simulink model "simulateAICENRobotInGazebo"  (R2022a)
settings: Solver=FixedStepAuto  StartTime=0.0  StopTime=inf  RelTol=1e-3
model workspace (MAT data in the model file):
  start = [2 8]
undefined symbols (not defined in the file or in its folder): avoidCollisionDistance, chargingStn, duration, effort, index, joint_name, left_wheel_clone_hinge, left_wheel_hinge, loadingStn, logicalMap, model_name, right_wheel_clone_hinge, right_wheel_hinge, scoutmini3, unloadingStn
libraries: robotgazebolib x19, robotalgslib x1, robotcorelib x1
settings Model: ParameterArgumentNames=start  Creator=The MathWorks, Inc.  LastModifiedBy=USER
settings SolverCC: AlgebraicLoopSolver=TrustRegion
settings DebuggingCC: UnconnectedInputMsg=warning  UnconnectedOutputMsg=warning  UnconnectedLineMsg=warning  ModelReferenceExtraNoncontSigs=none  SymbolicDimsDataTypeCodeGenerationDiagnostic=none  SFMachineParentedDataDiag=warning
settings RTWCC: DLArmComputeVersion=19.05

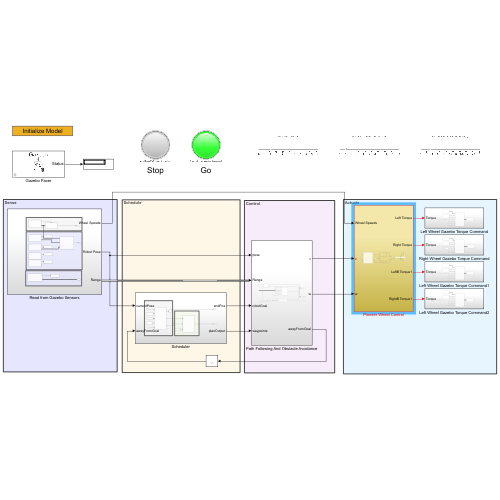
[thumbnail: Simulink's stored preview of the top-level diagram]
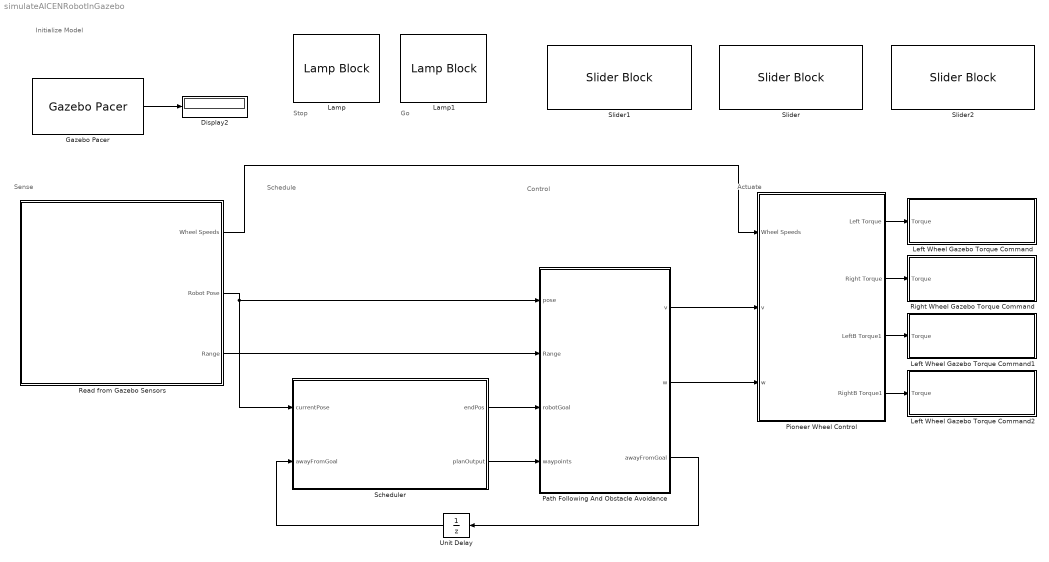
== system simulateAICENRobotInGazebo ==
  note: Actuate
  note: Control
  note: Schedule
  note: Sense
  note: Initialize Model
  note: Stop
  note: Go
  Display2 : Display
  Gazebo Pacer : robotgazebolib/Gazebo Pacer  ResetBehavior=Reset Gazebo simulation time and scene  SampleTime=0.01
      settings: SourceProductBaseCode=RO
  Lamp : LampBlock  LabelPosition=Bottom
  Lamp1 : LampBlock  LabelPosition=Bottom
  Left Wheel Gazebo Torque Command : Subsystem
  Left Wheel Gazebo Torque Command1 : Subsystem
  Left Wheel Gazebo Torque Command2 : Subsystem
  Path Following And Obstacle Avoidance : Subsystem
  Pioneer Wheel Control : Subsystem
  Read from Gazebo Sensors : Subsystem
  Right Wheel Gazebo Torque Command : Subsystem
  Scheduler : Subsystem
  Slider : SliderBlock  ScaleMax=10
  Slider1 : SliderBlock  ScaleMax=10
  Slider2 : SliderBlock  ScaleMax=5
  Unit Delay : UnitDelay  InitialCondition=1  SampleTime=-1  HasFrameUpgradeWarning=on
  wires:
  Read from Gazebo Sensors/2(Robot Pose) -> Scheduler/1(currentPose), Path Following And Obstacle Avoidance/1(pose)
  Pioneer Wheel Control/1(Left Torque) -> Left Wheel Gazebo Torque Command/1(Torque)
  Pioneer Wheel Control/2(Right Torque) -> Right Wheel Gazebo Torque Command/1(Torque)
  Read from Gazebo Sensors/1(Wheel Speeds) -> Pioneer Wheel Control/1(Wheel Speeds)
  Read from Gazebo Sensors/3(Range) -> Path Following And Obstacle Avoidance/2(Range)
  Path Following And Obstacle Avoidance/2(w) -> Pioneer Wheel Control/3(w)
  Gazebo Pacer/1 -> Display2/1
  Path Following And Obstacle Avoidance/3(awayFromGoal) -> Unit Delay/1
  Scheduler/1(endPos) -> Path Following And Obstacle Avoidance/3(robotGoal)
  Scheduler/2(planOutput) -> Path Following And Obstacle Avoidance/4(waypoints)
  Unit Delay/1 -> Scheduler/2(awayFromGoal)
  Path Following And Obstacle Avoidance/1(v) -> Pioneer Wheel Control/2(v)
  Pioneer Wheel Control/3(LeftB Torque1) -> Left Wheel Gazebo Torque Command1/1(Torque)
  Pioneer Wheel Control/4(RightB Torque1) -> Left Wheel Gazebo Torque Command2/1(Torque)

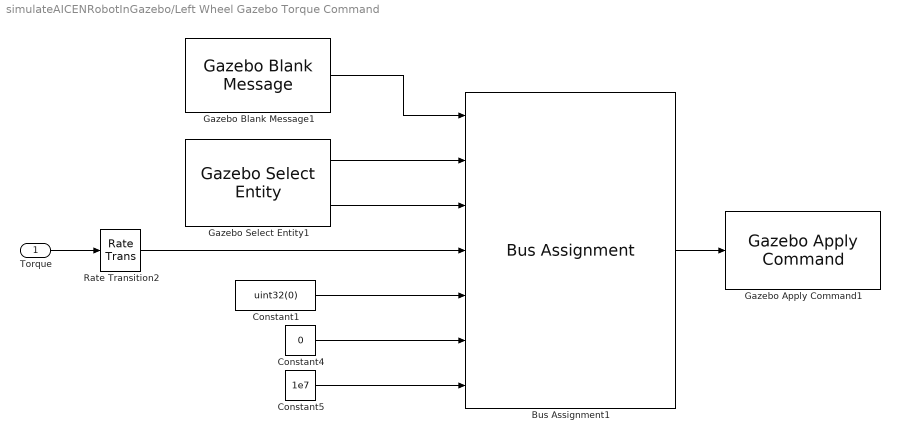
== system simulateAICENRobotInGazebo/Left Wheel Gazebo Torque Command ==
  Torque : Inport
  Bus Assignment1 : BusAssignment  AssignedSignals=model_name,joint_name,effort,index,duration.seconds,duration.nano_seconds
  Constant1 : Constant  Value=uint32(0)
  Constant4 : Constant  Value=0
  Constant5 : Constant  Value=1e7
  Gazebo Apply Command1 : robotgazebolib/Gazebo Apply Command  cmdType=ApplyJointTorque  sampleTime=0.01
      settings: SourceProductBaseCode=RO
  Gazebo Blank Message1 : robotgazebolib/Gazebo Blank Message  msgType=ApplyJointTorque  sampleTime=0.01  busName='Gazebo_SL_Bus_gazebo_msgs_ApplyJointTorque'
      settings: SourceProductBaseCode=RO
  Gazebo Select Entity1 : robotgazebolib/Gazebo Select Entity  modelElemName=scoutmini3/left_wheel_hinge  outputArraySize=128  OutputLabel=Joint  SelectType=Joint
      settings: SourceProductBaseCode=RO
  Rate Transition2 : RateTransition
  wires:
  Bus Assignment1/1 -> Gazebo Apply Command1/1
  Constant5/1 -> Bus Assignment1/7
  Gazebo Blank Message1/1 -> Bus Assignment1/1
  Gazebo Select Entity1/2 -> Bus Assignment1/3
  Gazebo Select Entity1/1 -> Bus Assignment1/2
  Torque/1 -> Rate Transition2/1
  Constant4/1 -> Bus Assignment1/6
  Rate Transition2/1 -> Bus Assignment1/4
  Constant1/1 -> Bus Assignment1/5

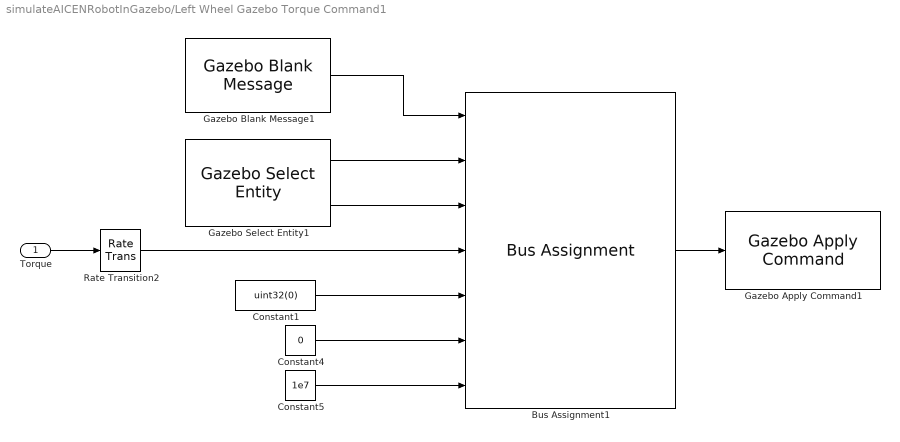
== system simulateAICENRobotInGazebo/Left Wheel Gazebo Torque Command1 ==
  Torque : Inport
  Bus Assignment1 : BusAssignment  AssignedSignals=model_name,joint_name,effort,index,duration.seconds,duration.nano_seconds
  Constant1 : Constant  Value=uint32(0)
  Constant4 : Constant  Value=0
  Constant5 : Constant  Value=1e7
  Gazebo Apply Command1 : robotgazebolib/Gazebo Apply Command  cmdType=ApplyJointTorque  sampleTime=0.01
      settings: SourceProductBaseCode=RO
  Gazebo Blank Message1 : robotgazebolib/Gazebo Blank Message  msgType=ApplyJointTorque  sampleTime=0.01  busName='Gazebo_SL_Bus_gazebo_msgs_ApplyJointTorque'
      settings: SourceProductBaseCode=RO
  Gazebo Select Entity1 : robotgazebolib/Gazebo Select Entity  modelElemName=scoutmini3/left_wheel_clone_hinge  outputArraySize=128  OutputLabel=Joint  SelectType=Joint
      settings: SourceProductBaseCode=RO
  Rate Transition2 : RateTransition
  wires:
  Bus Assignment1/1 -> Gazebo Apply Command1/1
  Constant5/1 -> Bus Assignment1/7
  Gazebo Blank Message1/1 -> Bus Assignment1/1
  Gazebo Select Entity1/2 -> Bus Assignment1/3
  Gazebo Select Entity1/1 -> Bus Assignment1/2
  Torque/1 -> Rate Transition2/1
  Constant4/1 -> Bus Assignment1/6
  Rate Transition2/1 -> Bus Assignment1/4
  Constant1/1 -> Bus Assignment1/5

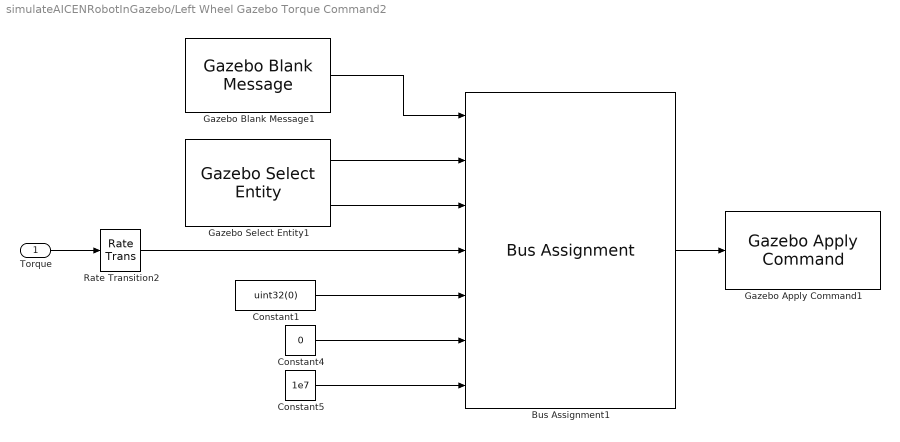
== system simulateAICENRobotInGazebo/Left Wheel Gazebo Torque Command2 ==
  Torque : Inport
  Bus Assignment1 : BusAssignment  AssignedSignals=model_name,joint_name,effort,index,duration.seconds,duration.nano_seconds
  Constant1 : Constant  Value=uint32(0)
  Constant4 : Constant  Value=0
  Constant5 : Constant  Value=1e7
  Gazebo Apply Command1 : robotgazebolib/Gazebo Apply Command  cmdType=ApplyJointTorque  sampleTime=0.01
      settings: SourceProductBaseCode=RO
  Gazebo Blank Message1 : robotgazebolib/Gazebo Blank Message  msgType=ApplyJointTorque  sampleTime=0.01  busName='Gazebo_SL_Bus_gazebo_msgs_ApplyJointTorque'
      settings: SourceProductBaseCode=RO
  Gazebo Select Entity1 : robotgazebolib/Gazebo Select Entity  modelElemName=scoutmini3/right_wheel_clone_hinge  outputArraySize=128  OutputLabel=Joint  SelectType=Joint
      settings: SourceProductBaseCode=RO
  Rate Transition2 : RateTransition
  wires:
  Bus Assignment1/1 -> Gazebo Apply Command1/1
  Constant5/1 -> Bus Assignment1/7
  Gazebo Blank Message1/1 -> Bus Assignment1/1
  Gazebo Select Entity1/2 -> Bus Assignment1/3
  Gazebo Select Entity1/1 -> Bus Assignment1/2
  Torque/1 -> Rate Transition2/1
  Constant4/1 -> Bus Assignment1/6
  Rate Transition2/1 -> Bus Assignment1/4
  Constant1/1 -> Bus Assignment1/5

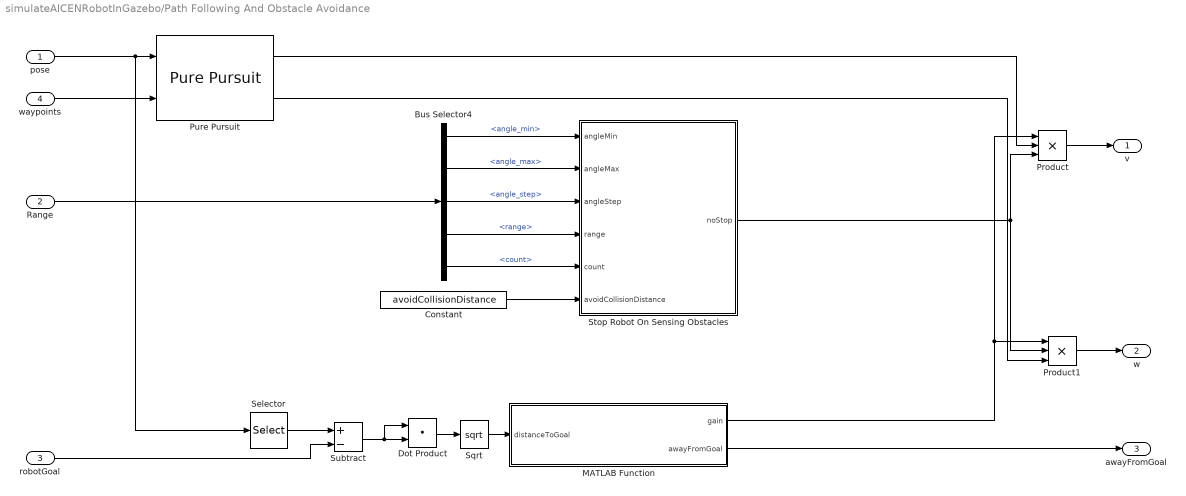
== system simulateAICENRobotInGazebo/Path Following And Obstacle Avoidance ==
  pose : Inport
  Range : Inport  Port=2
  robotGoal : Inport  Port=3
  waypoints : Inport  Port=4
  Bus Selector4 : BusSelector  OutputSignals=angle_min,angle_max,angle_step,range,count
  Constant : Constant  Value=avoidCollisionDistance
  Dot Product : DotProduct  OutDataTypeStr=Inherit: Inherit via internal rule
  MATLAB Function : MATLAB Function  TreatAsAtomicUnit=on
  Product : Product  Inputs=3
  Product1 : Product  Inputs=3
  Pure Pursuit : robotalgslib/Pure Pursuit  DesiredLinearVelocity=0.8  MaxAngularVelocity=1  LookaheadDistance=1  TargetDirPort=off  SimulateUsing=Code generation
  Selector : Selector  InputPortWidth=3  IndexOptions=Index vector (dialog)  Indices=[1 2]  OutputSizes=1
  Sqrt : Sqrt
  Stop Robot On Sensing Obstacles : MATLAB Function  TreatAsAtomicUnit=on
  Subtract : Sum  Inputs=+-
  v : Outport
  w : Outport  Port=2
  awayFromGoal : Outport  Port=3
  wires:
  Product1/1 -> w/1
  Product/1 -> v/1
  Stop Robot On Sensing Obstacles/1(noStop) -> Product/3, Product1/2
  Pure Pursuit/1 -> Product/2
  Pure Pursuit/2 -> Product1/3
  MATLAB Function/1(gain) -> Product/1, Product1/1
  Bus Selector4/4 -> Stop Robot On Sensing Obstacles/4(range)  "<range>"
  Range/1 -> Bus Selector4/1
  Constant/1 -> Stop Robot On Sensing Obstacles/6(avoidCollisionDistance)
  Bus Selector4/5 -> Stop Robot On Sensing Obstacles/5(count)  "<count>"
  Bus Selector4/1 -> Stop Robot On Sensing Obstacles/1(angleMin)  "<angle_min>"
  Bus Selector4/2 -> Stop Robot On Sensing Obstacles/2(angleMax)  "<angle_max>"
  Bus Selector4/3 -> Stop Robot On Sensing Obstacles/3(angleStep)  "<angle_step>"
  Sqrt/1 -> MATLAB Function/1(distanceToGoal)
  Subtract/1 -> Dot Product/1, Dot Product/2
  Selector/1 -> Subtract/1
  Dot Product/1 -> Sqrt/1
  robotGoal/1 -> Subtract/2
  MATLAB Function/2(awayFromGoal) -> awayFromGoal/1
  pose/1 -> Selector/1, Pure Pursuit/1
  waypoints/1 -> Pure Pursuit/2

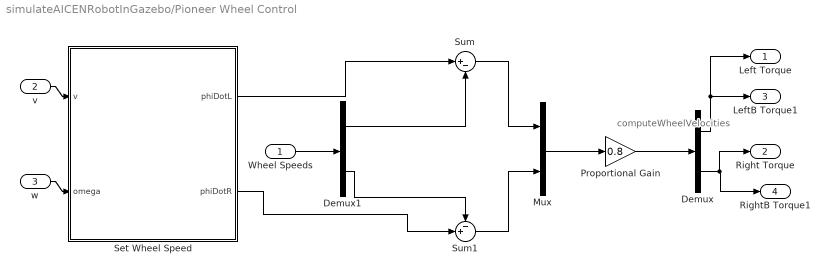
== system simulateAICENRobotInGazebo/Pioneer Wheel Control ==
  note: computeWheelVelocities
  Wheel Speeds : Inport
  v : Inport  Port=2
  w : Inport  Port=3
  Demux : Demux  Outputs=2
  Demux1 : Demux  Outputs=2
  Mux : Mux  Inputs=2
  Proportional Gain : Gain  Gain=0.8
  Set Wheel Speed : MATLAB Function  TreatAsAtomicUnit=on
  Sum : Sum  Inputs=|+-
  Sum1 : Sum  Inputs=-+|
  Left Torque : Outport
  Right Torque : Outport  Port=2
  LeftB Torque1 : Outport  Port=3
  RightB Torque1 : Outport  Port=4
  wires:
  Sum1/1 -> Mux/2
  Set Wheel Speed/1(phiDotL) -> Sum/1
  Sum/1 -> Mux/1
  Mux/1 -> Proportional Gain/1
  Proportional Gain/1 -> Demux/1
  Wheel Speeds/1 -> Demux1/1
  Demux1/1 -> Sum/2
  Set Wheel Speed/2(phiDotR) -> Sum1/2
  Demux1/2 -> Sum1/1
  v/1 -> Set Wheel Speed/1(v)
  w/1 -> Set Wheel Speed/2(omega)
  Demux/2 -> Right Torque/1, RightB Torque1/1
  Demux/1 -> LeftB Torque1/1, Left Torque/1

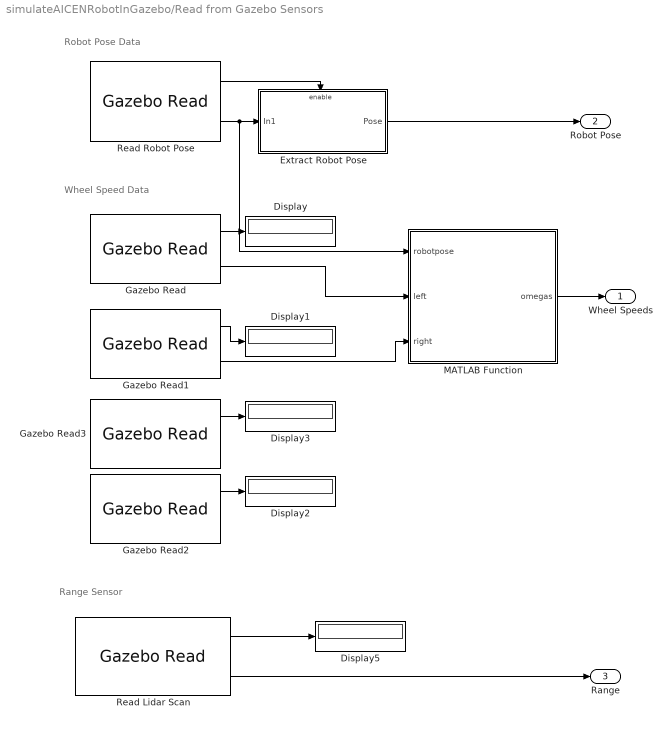
== system simulateAICENRobotInGazebo/Read from Gazebo Sensors ==
  note: Robot Pose Data
  note: Wheel Speed Data
  note: Range Sensor
  Display{,1..3,5} (5 alike) : Display
  Extract Robot Pose : Subsystem
  Gazebo Read : robotgazebolib/Gazebo Read  topicSource=Specify your own  topic=/gazebo/ground_truth/world_pose/scoutmini3/left_wheel  messageType=gazebo_msgs/Pose  sampleTime=0.01
      settings: SourceProductBaseCode=RO
  Gazebo Read1 : robotgazebolib/Gazebo Read  topicSource=Specify your own  topic=/gazebo/ground_truth/world_pose/scoutmini3/right_wheel  messageType=gazebo_msgs/Pose  sampleTime=0.01
      settings: SourceProductBaseCode=RO
  Gazebo Read2 : robotgazebolib/Gazebo Read  topicSource=Specify your own  topic=/gazebo/ground_truth/world_pose/scoutmini3/right_wheel_clone  messageType=gazebo_msgs/Pose  sampleTime=0.01
      settings: SourceProductBaseCode=RO
  Gazebo Read3 : robotgazebolib/Gazebo Read  topicSource=Specify your own  topic=/gazebo/ground_truth/world_pose/scoutmini3/left_wheel_clone  messageType=gazebo_msgs/Pose  sampleTime=0.01
      settings: SourceProductBaseCode=RO
  MATLAB Function : MATLAB Function  TreatAsAtomicUnit=on
  Read Lidar Scan : robotgazebolib/Gazebo Read  topicSource=Specify your own  topic=/gazebo/default/scoutmini3/hokuyo/link/laser/scan  messageType=gazebo_msgs/LaserScan  sampleTime=0.01
      settings: SourceProductBaseCode=RO
  Read Robot Pose : robotgazebolib/Gazebo Read  topicSource=Specify your own  topic=/gazebo/ground_truth/world_pose/scoutmini3/chassis  messageType=gazebo_msgs/Pose  sampleTime=0.01
      settings: SourceProductBaseCode=RO
  Wheel Speeds : Outport
  Robot Pose : Outport  Port=2
  Range : Outport  Port=3
  wires:
  Read Robot Pose/2 -> MATLAB Function/1(robotpose), Extract Robot Pose/1(In1)
  Extract Robot Pose/1(Pose) -> Robot Pose/1
  Read Robot Pose/1 -> Extract Robot Pose/Enable
  Gazebo Read/1 -> Display/1
  Gazebo Read1/1 -> Display1/1
  MATLAB Function/1(omegas) -> Wheel Speeds/1
  Gazebo Read/2 -> MATLAB Function/2(left)
  Gazebo Read1/2 -> MATLAB Function/3(right)
  Read Lidar Scan/1 -> Display5/1
  Read Lidar Scan/2 -> Range/1
  Gazebo Read2/1 -> Display2/1
  Gazebo Read3/1 -> Display3/1

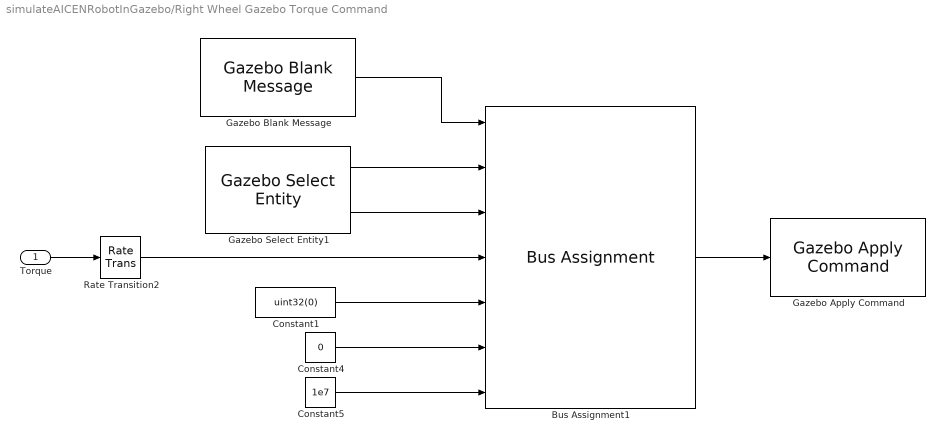
== system simulateAICENRobotInGazebo/Right Wheel Gazebo Torque Command ==
  Torque : Inport
  Bus Assignment1 : BusAssignment  AssignedSignals=model_name,joint_name,effort,index,duration.seconds,duration.nano_seconds
  Constant1 : Constant  Value=uint32(0)
  Constant4 : Constant  Value=0
  Constant5 : Constant  Value=1e7
  Gazebo Apply Command : robotgazebolib/Gazebo Apply Command  cmdType=ApplyJointTorque  sampleTime=0.01
      settings: SourceProductBaseCode=RO
  Gazebo Blank Message : robotgazebolib/Gazebo Blank Message  msgType=ApplyJointTorque  sampleTime=0.01  busName='Gazebo_SL_Bus_gazebo_msgs_ApplyJointTorque'
      settings: SourceProductBaseCode=RO
  Gazebo Select Entity1 : robotgazebolib/Gazebo Select Entity  modelElemName=scoutmini3/right_wheel_hinge  outputArraySize=128  OutputLabel=Joint  SelectType=Joint
      settings: SourceProductBaseCode=RO
  Rate Transition2 : RateTransition
  wires:
  Constant1/1 -> Bus Assignment1/5
  Rate Transition2/1 -> Bus Assignment1/4
  Constant4/1 -> Bus Assignment1/6
  Torque/1 -> Rate Transition2/1
  Gazebo Select Entity1/1 -> Bus Assignment1/2
  Gazebo Select Entity1/2 -> Bus Assignment1/3
  Gazebo Blank Message/1 -> Bus Assignment1/1
  Constant5/1 -> Bus Assignment1/7
  Bus Assignment1/1 -> Gazebo Apply Command/1

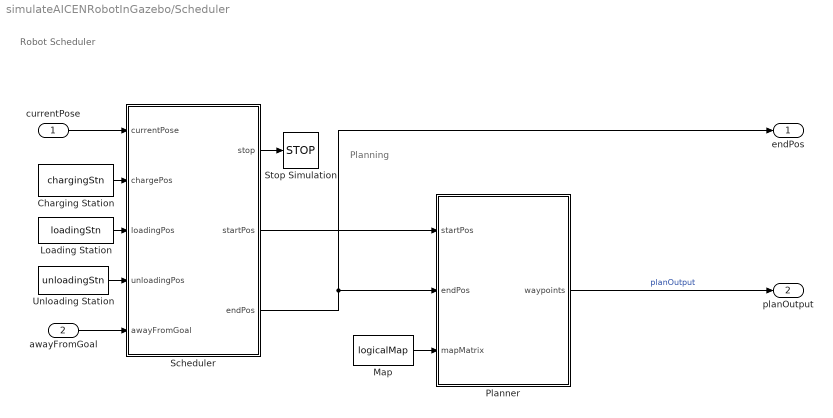
== system simulateAICENRobotInGazebo/Scheduler ==
  note: Planning
  note: Robot Scheduler
  currentPose : Inport
  awayFromGoal : Inport  Port=2
  "Charging Station " : Constant  Value=chargingStn  SampleTime=1
  Loading Station : Constant  Value=loadingStn
  "Map " : Constant  Value=logicalMap  SampleTime=1
  Planner : MATLAB Function  TreatAsAtomicUnit=on
  Scheduler : Stateflow chart  TreatAsAtomicUnit=on
  Stop Simulation : Stop
  Unloading Station : Constant  Value=unloadingStn  SampleTime=1
  endPos : Outport
  planOutput : Outport  Port=2
  wires:
  "Charging Station "/1 -> Scheduler/2(chargePos)
  Planner/1(waypoints) -> planOutput/1  "planOutput"
  Loading Station/1 -> Scheduler/3(loadingPos)
  currentPose/1 -> Scheduler/1(currentPose)
  Scheduler/1(stop) -> Stop Simulation/1
  Scheduler/2(startPos) -> Planner/1(startPos)
  Unloading Station/1 -> Scheduler/4(unloadingPos)
  "Map "/1 -> Planner/3(mapMatrix)
  Scheduler/3(endPos) -> endPos/1, Planner/2(endPos)
  awayFromGoal/1 -> Scheduler/5(awayFromGoal)

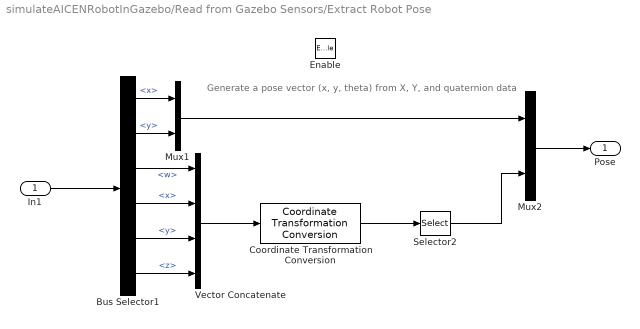
== system simulateAICENRobotInGazebo/Read from Gazebo Sensors/Extract Robot Pose ==
  note: Generate a pose vector (x, y, theta) from X, Y, and quaternion data
  In1 : Inport
  Enable : EnablePort
  Bus Selector1 : BusSelector  OutputSignals=position.x,position.y,orientation.w,orientation.x,orientation.y,orientation.z
  Coordinate Transformation Conversion : robotcorelib/Coordinate Transformation Conversion  InputRepresentation=Quaternion  InputEulerSequence=ZYX  ShowTrVecInputPort=on  OutputRepresentation=Euler Angles  OutputEulerSequence=ZYX  ShowTrVecOutputPort=on  SimulateUsing=Interpreted execution
      settings: SourceProductBaseCode=RO,NV,RR,UV
  Mux1 : Mux  Inputs=2
  Mux2 : Mux  Inputs=2
  Selector2 : Selector  InputPortWidth=3  IndexOptions=Index vector (dialog)  Indices=1  OutputSizes=1
  Vector Concatenate : Concatenate  NumInputs=4
  Pose : Outport  VectorParamsAs1DForOutWhenUnconnected=off
  wires:
  Vector Concatenate/1 -> Coordinate Transformation Conversion/1
  Coordinate Transformation Conversion/1 -> Selector2/1
  Mux1/1 -> Mux2/1
  Selector2/1 -> Mux2/2
  Mux2/1 -> Pose/1
  Bus Selector1/6 -> Vector Concatenate/4  "<z>"
  Bus Selector1/1 -> Mux1/1  "<x>"
  Bus Selector1/4 -> Vector Concatenate/2  "<x>"
  Bus Selector1/2 -> Mux1/2  "<y>"
  Bus Selector1/3 -> Vector Concatenate/1  "<w>"
  Bus Selector1/5 -> Vector Concatenate/3  "<y>"
  In1/1 -> Bus Selector1/1

== matlab function simulateAICENRobotInGazebo/Scheduler/Planner ==
  settings: updateMethod=DISCRETE
  data: startPos input size=[1 2]; endPos input size=[1 2]; waypoints output size=[150 2]; mapMatrix input; mapScalingFactor parameter
function waypoints = planning(startPos, endPos, mapMatrix, mapScalingFactor)

persistent waypointsInternal
persistent prevStartPos
persistent prevEndPos

% Set constant parameters
maxNumNodes = 150;

% Initialize persistent variables that are used downstream
%다운스트림에서 사용되는 영구 변수 초기화
if isempty(prevStartPos)
    prevStartPos = startPos;
end

if isempty(prevEndPos)
    prevEndPos = endPos;
end

isNewPath = (~isequal(prevStartPos, startPos) || ~isequal(prevEndPos, endPos));

if isempty(waypointsInternal) || isNewPath
    % Two conditions in which waypoints must be set: they are not yet
    % initialized, or they are initialized, but the current start and end
    % do not match those used to generate the previous set of waypoints
    %웨이포인트를 설정해야 하는 두 가지 조건: 아직 초기화되지 않았거나 초기화되었지만 현재 시작과 끝이 이전 웨이포인트 세트를 생성하는 데 사용된 조건과 일치하지 않습니다.
    [waypointsInternal] = planPath(mapMatrix, maxNumNodes, startPos, endPos, mapScalingFactor);
end

% Update the outputs
waypoints = waypointsInternal;

% Update the persistent variables that indicate previous state
%이전 상태를 나타내는 영구 변수 업데이트
prevStartPos = startPos;
prevEndPos = endPos;

%% Helper Function

function wayPoints = planPath(mapMatrix, maxNodes, startPos, endPos, mapScalingFactor)
    
    % Create a probabilistic roadmap 확률적 로드맵 설정
    map = binaryOccupancyMap(mapMatrix, mapScalingFactor);
    prm = mobileRobotPRM(map, maxNodes);
    
    % Find a path between two points
    xy = findpath(prm, startPos(:)', endPos(:)');
    wayPoints = repmat(endPos(:)', maxNodes, 1);
    
    % Number of nodes that are actually used
    numNodes = length(xy);
    wayPoints(1:numNodes,:) = xy;    

end

end

== matlab function simulateAICENRobotInGazebo/Pioneer Wheel Control/Set Wheel Speed ==
  data: v input; omega input; phiDotL output; phiDotR output
function [phiDotL, phiDotR]= wheelSpeed(v, omega)  %phiDotBL,phiDotBR] = wheelSpeed(v, omega)
%%wheelSpeed computes the speed of the left and the right wheel given the linear and angular velocities.

% Robot's constants
trackWidth = 0.490;
wheelRadius = 0.175/2;

% Convert velocity and heading angular velocity to wheel speeds
phiDotL = (v - trackWidth/10*omega)/wheelRadius;
phiDotR = (v + trackWidth/10*omega)/wheelRadius;  %기본값 2인데 회전을너무 안해서 변경해보는중 
%phiDotBL = (v - trackWidth/4*omega)/wheelRadius;
%phiDotBR = (v + trackWidth/4*omega)/wheelRadius;



end

== stateflow chart simulateAICENRobotInGazebo/Scheduler/Scheduler ==
  settings: sampleTime=0.01
  state Loading
    entry,during:
    endPos = loadingPos';
  state Unloading
    entry, during:
    endPos = unloadingPos';
  state Charging
    entry, during:
    endPos = chargePos';
  state Stop
    entry:
    stop = true;
  (default) -> Loading : {startPos = chargePos';}
  Loading -> Unloading : [~awayFromGoal && after(stopDelay, tick)]
      | {startPos = currentPose(1:2)';}
  Unloading -> Charging : [~awayFromGoal  && after(stopDelay, tick)]
      | {startPos = currentPose(1:2)';}
  Charging -> Stop : [~awayFromGoal]
  data: currentPose input; stop output =false; chargePos input size=[2 1]; loadingPos input size=[2 1]; unloadingPos input size=[2 1]; startPos output size=[1, 2]; endPos output size=[1, 2]; awayFromGoal input; stopDelay local =1.5 * 1e3

== matlab function simulateAICENRobotInGazebo/Read from Gazebo Sensors/MATLAB Function ==
  data: robotpose input; omegas output; left input; right input
function omegas = computeWheelVelocities(robotpose, left, right) %, bright, bleft) %(robotpose, left, right)
%computeWheelVelocities computes wheel velocity based on rate of change of
%the yaw angle of the wheel relative to its original mount on the robot
%body
%Compute Wheel Velocities는 로봇의 원래 마운트를 기준으로 휠의 요 각도 변화율을 기반으로 휠 속도를 계산합니다.

persistent initAngles
if isempty(initAngles)
    initAngles = zeros(2,1);
end
sampleTime = 0.01;

% compute rotation between wheel original mount on the robot body and world
% frame
%로봇 본체의 휠 원래 마운트와 월드 프레임 사이의 회전 계산
robotRtom = quat2rotm([robotpose.orientation.w, robotpose.orientation.x, robotpose.orientation.y, robotpose.orientation.z]);
originalWheelMount = robotRtom*eul2rotm([pi/2 pi/2 0]);

% get rotation between wheel and the world frame
%휠과 월드 프레임 사이의 회전을 얻습니다.
leftRtom = quat2rotm([left.orientation.w, left.orientation.x, left.orientation.y, left.orientation.z]);
rightRtom = quat2rotm([right.orientation.w, right.orientation.x, right.orientation.y, right.orientation.z]);

%BleftRtom = quat2rotm([bleft.orientation.w, bleft.orientation.x, bleft.orientation.y, bleft.orientation.z]); %테스트용
%BrightRtom = quat2rotm([bright.orientation.w, bright.orientation.x, bright.orientation.y, bright.orientation.z]);


% compute relative rotation between wheel and its original mount
%휠과 원래 마운트 사이의 상대 회전 계산
leftRotation = rotm2eul(originalWheelMount'*leftRtom);
rightRotation = rotm2eul(originalWheelMount'*rightRtom);

%BleftRotation = rotm2eul(originalWheelMount'*BleftRtom);
%BrightRotation = rotm2eul(originalWheelMount'*BrightRtom);

% compute angluar velocity using the angle difference between the current
% angle pose and the the angle pose in last time step
%현재 각도 포즈와 마지막 시간 단계의 각도 포즈 사이의 각도 차이를 사용하여 각 속도를 계산합니다.
angles = [leftRotation(1); rightRotation(1)];
omegas = angdiff(initAngles, angles)/sampleTime;
initAngles = angles;

== matlab function simulateAICENRobotInGazebo/Path Following And Obstacle Avoidance/MATLAB Function ==
  data: distanceToGoal input; gain output; awayFromGoal output
function [gain, awayFromGoal] = slowDownNearGoal(distanceToGoal)
%%slowDownNearGoal gradually slows the robot when it reaches a goal location.
%slowDownNearGoal은 로봇이 목표 위치에 도달하면 점차적으로 로봇의 속도를 늦춥니다.

%continue to move at the normal angular and linear velocity
%정상 각 및 선형 속도로 계속 이동
gain = 1;

%assume that the robot is away from goal
%로봇이 목표에서 멀리 떨어져 있다고 가정
awayFromGoal = 1;

%threshold to determine if the robot has reached the goal
%로봇이 목표에 도달했는지 판단하기 위한 임계값
atGoalThreshold = 0.5;
slowThreshold = 1;

%if the robot is within range and should start slowing down
%로봇이 범위 내에 있고 감속을 시작해야 하는 경우
if(distanceToGoal < slowThreshold)
    
    %speed reduction gain
    gain = distanceToGoal / slowThreshold;
    if(distanceToGoal < atGoalThreshold)
        %stop the robot entirely
        gain = 0;
        %the robot has reached the goal
        awayFromGoal = 0;
    end
end

== matlab function simulateAICENRobotInGazebo/Path Following And Obstacle Avoidance/Stop Robot On Sensing Obstacles ==
  data: angleMin input; angleMax input; angleStep input; range input; count input; noStop output size=1; avoidCollisionDistance input
function noStop= stopRobot(angleMin, angleMax, angleStep, range, count, avoidCollisionDistance)
%%stopRobot stops the robot based on the range sensor.  
%   The robot has an on-board range sensor which it uses to detect
%   obstacles. 

%limits on the angle of range readings for defining viewing scope of the robot
%로봇의 시야범위각도 설정 
angMin = -pi/10;
angMax = pi/10;

%signal the robot to continue moving unless it sees an obstacle
%장애물이 보이지 않는 한 로봇이 계속 움직이도록 신호를 보냅니다.
noStop = true;

%if the ray count is non-zero
if count ~= 0
    %create a lidar scan object from the range readings
    %범위 판독값에서 라이더 스캔 개체 생성
    scan = lidarScan(range, angleMin:angleStep:angleMax);
    
    %filter out non-zero ranges which are in robot's scope. Range-values are zero if
    %there are no obstacles.
    %로봇의 범위에 있는 0이 아닌 범위를 필터링합니다. 장애물이 없는 경우 범위 값은 0입니다.
    rangeScope = scan.Ranges((scan.Angles > angMin) & ... 
                            (scan.Angles < angMax) & ...
                            (scan.Ranges ~= 0));
                        
    %signal the robot to continue to move if none of the ranges are less than 2m
    %범위가 2m 미만인 경우 로봇이 계속 움직이도록 신호를 보냅니다.
    noStop = ~any(rangeScope < avoidCollisionDistance);
end

end
